simulink model "EvPowertrainController2EM"  (R2024a)
settings: configuration reference "VehicleFixed10ms" (kept outside this file)
model workspace (MAT data in the model file):
  CtrlVcuAccelPdlBpts = [0 0.8 1]
  CtrlVcuBattPnlty = 10000000
  CtrlVcuBattSOCBpts = [0 20 60 80 100]
  CtrlVcuCnstrntPnltyFctr = 10000000
  CtrlVcuEMPnlty = 100
  CtrlVcuEMTrqSplitGrid = 200
  CtrlVcuFallRate = -500
  CtrlVcuMaxAccelG = 1
  CtrlVcuMaxDecelG = -1.5
  CtrlVcuPwrDeltaPnlty = 50
  CtrlVcuPwrRatePnlty = [25 25 100]
  CtrlVcuRiseRate = 500
  CtrlVcuRoadMuEst = 0.8
  CtrlVcuSftyFctr = 0.9
  CtrlVcuTracPwrErrPnlty = 25
  CtrlVcuTrqVecBrkThresh = 0.01
  CtrlVcuTrqVecIGain = 0
  CtrlVcuTrqVecMinTrq = 25
  CtrlVcuTrqVecPGain = -2000
  CtrlVcuTrqVecSteerThresh = 0.349065850399
  CtrlVcuTrqVecVelThresh = 2.5
  N_P0 = 3
undefined symbols (not defined in the file): CtrlBcuTrlrBrkGain, CtrlVcuEvChrgLmtBpt, CtrlVcuEvRegenBrkCutOff, CtrlVcuEvRegenBrkSpdBpt, CtrlVcuEvSocBpt, eff, EnvGrvty, PlntBrkActrBoreFrnt, PlntBrkFrntBias, PlntBrkKinFricCffFrnt, PlntBrkNumPadsFrnt, PlntBrkPadMeanRadiusFrnt, PlntBrkPrsFctr, PlntBrkRearBias, PlntDiffrntl2Eff, PlntDiffrntl2Ratio, PlntDiffrntlEff, PlntDiffrntlRatio, PlntEM1EffTbl, PlntEM1Spd, PlntEM1SpdEff, PlntEM1Trq, PlntEM1TrqEff, PlntEM2EffTbl, PlntEM2Spd, PlntEM2SpdEff, PlntEM2Trq, PlntEM2TrqEff, PlntEM3EffTbl, PlntEM3Spd, PlntEM3SpdEff, PlntEM3Trq, PlntEM3TrqEff, PlntEMWhlGearEffFL, PlntEMWhlGearEffRL, PlntEMWhlGearRatioFL, PlntEMWhlGearRatioRL, PlntTransEffSpdBpt, PlntTransEffTbl, PlntTransEffTempBpt, PlntTransEffTrqBpt, PlntTransGearNumVect, PlntTransGearRatioVect, PlntVehCGHgtAxl, PlntVehDstCGFrntAxl, PlntVehDstCGRearAxl, PlntVehMass, PlntWhlLdRadius
libraries: simulink x16, autolibutils x2, slpidlib x2
(part 2 of 5)

== system EvPowertrainController2EM/Energy Management/Calculate Average EMSpd and Wheel Torque Curves for Front and Rear Axles/3EM Dual Front ==
  note: Calculate average speed
      | of EMs on axle
  note: Reflect EMTrq to WhlTrq
      | due to possible gearing
      | differences
  EMSpd : Inport
  Gear : Inport  Port=2
  EMTrq2WhlTrqFrnt : Subsystem  Variant=on  VariantControlMode=label  VariantControl=1  LabelModeActiveChoice=3
  EMTrq2WhlTrqRear : Subsystem  Variant=on  VariantControlMode=label  VariantControl=1  LabelModeActiveChoice=3
  Gain : Gain  Gain=1/2
  Maximum Torque Front Axle : Subsystem
  Maximum Torque Rear Axle : Subsystem
  Selector : Selector  InputPortWidth=3  IndexOptions=Index vector (dialog)  Indices=[1 2]  OutputSizes=1
  Selector1 : Selector  InputPortWidth=3  IndexOptions=Index vector (dialog)  Indices=[3]  OutputSizes=1
  Sum of Elements : Sum  Inputs=+
  Vector Concatenate : Concatenate
  Vector Concatenate1 : Concatenate
  EMAvgSpdVec : Outport
  WhlTrqMaxVec : Outport  Port=2
  wires:
  Selector/1 -> Sum of Elements/1
  EMSpd/1 -> Selector1/1, Selector/1
  Sum of Elements/1 -> Gain/1
  Maximum Torque Rear Axle/1(EMTrq) -> EMTrq2WhlTrqRear/2(EMTrqCmd)
  Maximum Torque Front Axle/1(EMTrq) -> EMTrq2WhlTrqFrnt/2(EMTrqCmd)
  Gain/1 -> Vector Concatenate1/1, EMTrq2WhlTrqFrnt/3(EMSpd), Maximum Torque Front Axle/1(EMSpd)
  Gear/1 -> EMTrq2WhlTrqRear/1(Gear), EMTrq2WhlTrqFrnt/1(Gear)
  Selector1/1 -> Maximum Torque Rear Axle/1(EMSpd), EMTrq2WhlTrqRear/3(EMSpd), Vector Concatenate1/2
  EMTrq2WhlTrqRear/1(WhlMotTrq) -> Vector Concatenate/2
  EMTrq2WhlTrqFrnt/1(WhlMotTrq) -> Vector Concatenate/1
  Vector Concatenate/1 -> WhlTrqMaxVec/1
  Vector Concatenate1/1 -> EMAvgSpdVec/1

== system EvPowertrainController2EM/Energy Management/Calculate Average EMSpd and Wheel Torque Curves for Front and Rear Axles/3EM Dual Rear ==
  note: Calculate average speed
      | of EMs on axle
  note: Reflect EMTrq to WhlTrq
      | due to possible gearing
      | differences
  EMSpd : Inport
  Gear : Inport  Port=2
  EMTrq2WhlTrqFrnt : Subsystem  Variant=on  VariantControlMode=label  VariantControl=1  LabelModeActiveChoice=3
  EMTrq2WhlTrqRear : Subsystem  Variant=on  VariantControlMode=label  VariantControl=1  LabelModeActiveChoice=3
  Gain : Gain  Gain=1/2
  Maximum Torque Front Axle : Subsystem
  Maximum Torque Rear Axle : Subsystem
  Selector : Selector  InputPortWidth=3  IndexOptions=Index vector (dialog)  Indices=[2 3]  OutputSizes=1
  Selector1 : Selector  InputPortWidth=3  IndexOptions=Index vector (dialog)  Indices=[1]  OutputSizes=1
  Sum of Elements : Sum  Inputs=+
  Vector Concatenate : Concatenate
  Vector Concatenate1 : Concatenate
  EMAvgSpdVec : Outport
  WhlTrqMaxVec : Outport  Port=2
  wires:
  Sum of Elements/1 -> Gain/1
  EMSpd/1 -> Selector1/1, Selector/1
  Selector/1 -> Sum of Elements/1
  EMTrq2WhlTrqRear/1(WhlMotTrq) -> Vector Concatenate/2
  Gain/1 -> Vector Concatenate1/2, EMTrq2WhlTrqRear/3(EMSpd), Maximum Torque Rear Axle/1(EMSpd)
  Maximum Torque Rear Axle/1(EMTrq) -> EMTrq2WhlTrqRear/2(EMTrqCmd)
  Maximum Torque Front Axle/1(EMTrq) -> EMTrq2WhlTrqFrnt/2(EMTrqCmd)
  Selector1/1 -> Vector Concatenate1/1, EMTrq2WhlTrqFrnt/3(EMSpd), Maximum Torque Front Axle/1(EMSpd)
  Gear/1 -> EMTrq2WhlTrqFrnt/1(Gear), EMTrq2WhlTrqRear/1(Gear)
  EMTrq2WhlTrqFrnt/1(WhlMotTrq) -> Vector Concatenate/1
  Vector Concatenate/1 -> WhlTrqMaxVec/1
  Vector Concatenate1/1 -> EMAvgSpdVec/1

== system EvPowertrainController2EM/Energy Management/Calculate Average EMSpd and Wheel Torque Curves for Front and Rear Axles/4EM ==
  note: Calculate average speed
      | of EMs on axle
  note: Reflect EMTrq to WhlTrq
      | due to possible gearing
      | differences
  EMSpd : Inport
  Gear : Inport  Port=2
  EMTrq2WhlTrqFrnt : Subsystem  Variant=on  VariantControlMode=label  VariantControl=1  LabelModeActiveChoice=3
  EMTrq2WhlTrqRear : Subsystem  Variant=on  VariantControlMode=label  VariantControl=1  LabelModeActiveChoice=3
  Gain : Gain  Gain=1/2
  Gain1 : Gain  Gain=1/2
  Maximum Torque Front Axle : Subsystem
  Maximum Torque Rear Axle : Subsystem
  Selector : Selector  InputPortWidth=4  IndexOptions=Index vector (dialog)  Indices=[3 4]  OutputSizes=1
  Selector1 : Selector  InputPortWidth=4  IndexOptions=Index vector (dialog)  Indices=[1 2]  OutputSizes=1
  Sum of Elements : Sum  Inputs=+
  Sum of Elements1 : Sum  Inputs=+
  Vector Concatenate : Concatenate
  Vector Concatenate1 : Concatenate
  EMAvgSpdVec : Outport
  WhlTrqMaxVec : Outport  Port=2
  wires:
  Selector/1 -> Sum of Elements/1
  Selector1/1 -> Sum of Elements1/1
  EMSpd/1 -> Selector/1, Selector1/1
  Sum of Elements/1 -> Gain/1
  Sum of Elements1/1 -> Gain1/1
  EMTrq2WhlTrqRear/1(WhlMotTrq) -> Vector Concatenate/2
  Maximum Torque Front Axle/1(EMTrq) -> EMTrq2WhlTrqFrnt/2(EMTrqCmd)
  Maximum Torque Rear Axle/1(EMTrq) -> EMTrq2WhlTrqRear/2(EMTrqCmd)
  Gain1/1 -> Vector Concatenate1/1, EMTrq2WhlTrqFrnt/3(EMSpd), Maximum Torque Front Axle/1(EMSpd)
  EMTrq2WhlTrqFrnt/1(WhlMotTrq) -> Vector Concatenate/1
  Gear/1 -> EMTrq2WhlTrqRear/1(Gear), EMTrq2WhlTrqFrnt/1(Gear)
  Gain/1 -> Vector Concatenate1/2, Maximum Torque Rear Axle/1(EMSpd), EMTrq2WhlTrqRear/3(EMSpd)
  Vector Concatenate/1 -> WhlTrqMaxVec/1
  Vector Concatenate1/1 -> EMAvgSpdVec/1

== system EvPowertrainController2EM/Energy Management/Control Domain /Front Axle EM Torque Vector ==
  EMAvgSpdVec : Inport
  2EM or 3EM Dual Rear : Subsystem  VariantControl=2EM or 3EM Dual Rear
  3EM Dual Front or 4EM : Subsystem  VariantControl=3EM Dual Front or 4EM
  WhlEMFrntVecPos : Outport
  WhlEMFrntVecNeg : Outport  Port=2

== system EvPowertrainController2EM/Energy Management/Control Domain /Rear Axle EM Torque Vector ==
  EMAvgSpdVec : Inport
  2EM or 3EM Dual Front : Subsystem  VariantControl=2EM or 3EM Dual Front
  3EM Dual Rear or 4EM : Subsystem  VariantControl=3EM Dual Rear or 4EM
  WhlEMRearVecPos : Outport
  WhlEMRearVecNeg : Outport  Port=2

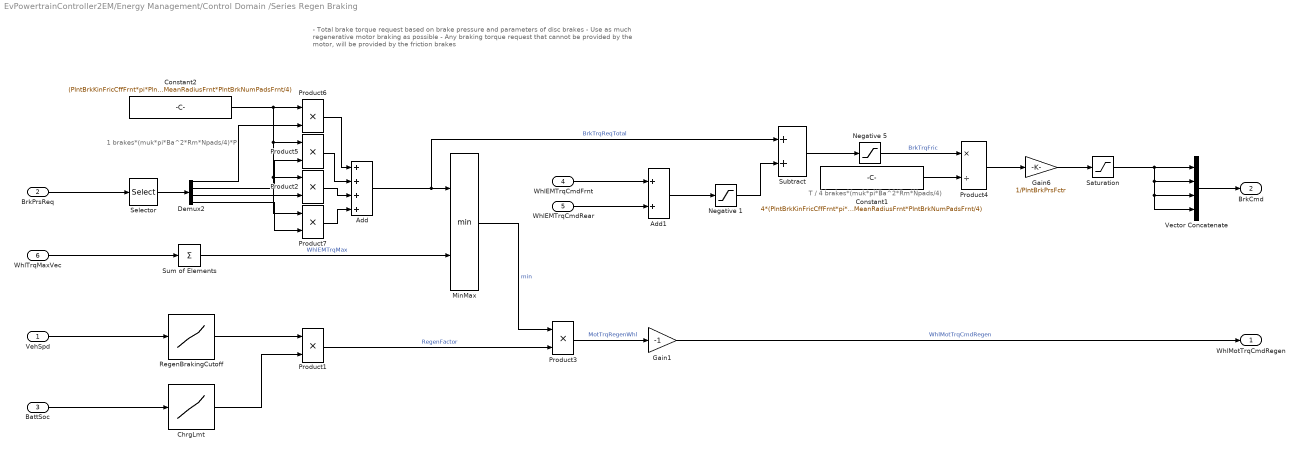
== system EvPowertrainController2EM/Energy Management/Control Domain /Series Regen Braking ==
  note: - Total brake torque request based on brake pressure and parameters of disc brakes
      | - Use as much regenerative motor braking as possible
      | - Any braking torque request that cannot be provided by the motor, will be provided by the friction brakes
  note: T / 4 brakes*(muk*pi*Ba^2*Rm*Npads/4)
  note: 1 brakes*(muk*pi*Ba^2*Rm*Npads/4)*P
  VehSpd : Inport
  "BrkPrsReq " : Inport  Port=2
  BattSoc : Inport  Port=3
  WhlEMTrqCmdFrnt : Inport  Port=4
  WhlEMTrqCmdRear : Inport  Port=5
  WhlTrqMaxVec : Inport  Port=6
  Add : Sum  Inputs=++++
  Add1 : Sum
  ChrgLmt : Lookup_n-D  NumberOfTableDimensions=1  BreakpointsForDimension1=CtrlVcuEvSocBpt  Table=CtrlVcuEvChrgLmtBpt  ExtrapMethod=Clip  UseLastTableValue=on  InternalRulePriority=Speed  RndMeth=Simplest
  Constant1 : Constant  Value=4*(PlntBrkKinFricCffFrnt*pi*PlntBrkActrBoreFrnt^2*PlntBrkPadMeanRadiusFrnt*PlntBrkNumPadsFrnt/4)
  Constant2 : Constant  Value=(PlntBrkKinFricCffFrnt*pi*PlntBrkActrBoreFrnt^2*PlntBrkPadMeanRadiusFrnt*PlntBrkNumPadsFrnt/4)
  Demux2 : Demux
  Gain1 : Gain  Gain=-1
  Gain6 : Gain  Gain=1/PlntBrkPrsFctr
  MinMax : MinMax  Inputs=2
  Negative 1 : Saturate  UpperLimit=0  LowerLimit=-inf
  Negative 5 : Saturate  UpperLimit=inf  LowerLimit=0
  Product{1..3,5..7} (6 alike) : Product
  Product4 : Product  Inputs=*/
  RegenBrakingCutoff : Lookup_n-D  NumberOfTableDimensions=1  BreakpointsForDimension1=CtrlVcuEvRegenBrkSpdBpt  Table=CtrlVcuEvRegenBrkCutOff  ExtrapMethod=Clip  UseLastTableValue=on  InternalRulePriority=Speed  RndMeth=Simplest
  Saturation : Saturate  UpperLimit=1  LowerLimit=0
  Selector : Selector  InputPortWidth=4  IndexOptions=Index vector (dialog)  Indices=[1 2 3 4]  OutputSizes=1
  Subtract : Sum
  Sum of Elements : Sum  Inputs=+
  Vector Concatenate : Concatenate  NumInputs=4
  " WhlMotTrqCmdRegen" : Outport  VectorParamsAs1DForOutWhenUnconnected=off
  " BrkCmd" : Outport  Port=2  VectorParamsAs1DForOutWhenUnconnected=off
  wires:
  Constant1/1 -> Product4/2
  MinMax/1 -> Product3/1  "min"
  ChrgLmt/1 -> Product1/2
  VehSpd/1 -> RegenBrakingCutoff/1
  RegenBrakingCutoff/1 -> Product1/1
  Product1/1 -> Product3/2  "RegenFactor"
  Subtract/1 -> Negative 5/1
  BattSoc/1 -> ChrgLmt/1
  Negative 5/1 -> Product4/1  "BrkTrqFric"
  Sum of Elements/1 -> MinMax/2  "WhlEMTrqMax"
  Demux2/2 -> Product5/2
  Demux2/1 -> Product6/2
  Selector/1 -> Demux2/1
  Product6/1 -> Add/1
  Product5/1 -> Add/2
  Add/1 -> Subtract/1, MinMax/1  "BrkTrqReqTotal"
  "BrkPrsReq "/1 -> Selector/1
  Vector Concatenate/1 -> " BrkCmd"/1
  Gain6/1 -> Saturation/1
  Product4/1 -> Gain6/1
  Saturation/1 -> Vector Concatenate/3, Vector Concatenate/4, Vector Concatenate/2, Vector Concatenate/1
  WhlTrqMaxVec/1 -> Sum of Elements/1
  Gain1/1 -> " WhlMotTrqCmdRegen"/1  "WhlMotTrqCmdRegen"
  Product3/1 -> Gain1/1  "MotTrqRegenWhl"
  Add1/1 -> Negative 1/1
  Negative 1/1 -> Subtract/2
  Product2/1 -> Add/3
  Product7/1 -> Add/4
  Demux2/3 -> Product2/2
  Demux2/4 -> Product7/2
  Constant2/1 -> Product7/1, Product2/1, Product5/1, Product6/1
  WhlEMTrqCmdFrnt/1 -> Add1/1
  WhlEMTrqCmdRear/1 -> Add1/2

== system EvPowertrainController2EM/Energy Management/Convert Whl to EMTrq Vector/2EM ==
  WhlEMTrqCmdFrnt : Inport
  WhlEMTrqCmdRear : Inport  Port=2
  EMAvgSpdVec : Inport  Port=3
  Diff Eta : Subsystem
  Diff Eta1 : Subsystem
  Divide1 : Product  Inputs=/*
  Divide2 : Product  Inputs=/*
  Gain1 : Gain  Gain=1/PlntDiffrntl2Ratio
  Gain3 : Gain  Gain=1/PlntDiffrntlRatio
  Selector : Selector  InputPortWidth=2  IndexOptions=Index vector (dialog)  Indices=[1]  OutputSizes=1
  Selector1 : Selector  InputPortWidth=2  IndexOptions=Index vector (dialog)  Indices=[2]  OutputSizes=1
  Unit Delay : UnitDelay  SampleTime=-1  HasFrameUpgradeWarning=on
  Unit Delay1 : UnitDelay  SampleTime=-1  HasFrameUpgradeWarning=on
  Vector Concatenate1 : Concatenate
  EMTrqCmd : Outport
  wires:
  WhlEMTrqCmdRear/1 -> Gain1/1
  Gain3/1 -> Divide2/2
  Divide2/1 -> Vector Concatenate1/1, Unit Delay/1
  WhlEMTrqCmdFrnt/1 -> Gain3/1
  Selector/1 -> Diff Eta/1(SpdIn)
  Unit Delay/1 -> Diff Eta/2(TrqIn)
  Diff Eta/1(eta) -> Divide2/1
  Diff Eta1/1(eta) -> Divide1/1
  Unit Delay1/1 -> Diff Eta1/2(TrqIn)
  Divide1/1 -> Unit Delay1/1, Vector Concatenate1/2
  Gain1/1 -> Divide1/2
  EMAvgSpdVec/1 -> Selector1/1, Selector/1
  Selector1/1 -> Diff Eta1/1(SpdIn)
  Vector Concatenate1/1 -> EMTrqCmd/1

== system EvPowertrainController2EM/Energy Management/Convert Whl to EMTrq Vector/3EM Dual Front ==
  WhlEMTrqCmdFrnt : Inport
  WhlEMTrqCmdRear : Inport  Port=2
  EMAvgSpdVec : Inport  Port=3
  Diff Eta : Subsystem
  Divide1 : Product  Inputs=/*
  Divide2 : Product  Inputs=/*
  Dual EMs : Gain  Gain=1/2
  Gain1 : Gain  Gain=1/PlntDiffrntl2Ratio
  Gain3 : Gain  Gain=1/PlntEMWhlGearRatioFL
  Gear Eta : Subsystem
  Selector : Selector  InputPortWidth=2  IndexOptions=Index vector (dialog)  Indices=[1]  OutputSizes=1
  Selector1 : Selector  InputPortWidth=2  IndexOptions=Index vector (dialog)  Indices=[2]  OutputSizes=1
  Unit Delay : UnitDelay  SampleTime=-1  HasFrameUpgradeWarning=on
  Unit Delay1 : UnitDelay  SampleTime=-1  HasFrameUpgradeWarning=on
  Vector Concatenate : Concatenate  NumInputs=3
  EMTrqCmd : Outport
  wires:
  Selector1/1 -> Diff Eta/1(SpdIn)
  EMAvgSpdVec/1 -> Selector/1, Selector1/1
  Gain1/1 -> Divide1/2
  Unit Delay1/1 -> Diff Eta/2(TrqIn)
  Diff Eta/1(eta) -> Divide1/1
  Gear Eta/1(eta) -> Divide2/1
  Unit Delay/1 -> Gear Eta/2(TrqIn)
  Selector/1 -> Gear Eta/1(SpdIn)
  WhlEMTrqCmdFrnt/1 -> Dual EMs/1
  Gain3/1 -> Divide2/2
  WhlEMTrqCmdRear/1 -> Gain1/1
  Divide1/1 -> Vector Concatenate/3, Unit Delay1/1
  Vector Concatenate/1 -> EMTrqCmd/1
  Divide2/1 -> Vector Concatenate/1, Vector Concatenate/2, Unit Delay/1
  Dual EMs/1 -> Gain3/1

== system EvPowertrainController2EM/Energy Management/Convert Whl to EMTrq Vector/3EM Dual Rear ==
  WhlEMTrqCmdFrnt : Inport
  WhlEMTrqCmdRear : Inport  Port=2
  EMAvgSpdVec : Inport  Port=3
  Diff Eta : Subsystem
  Divide1 : Product  Inputs=/*
  Divide2 : Product  Inputs=/*
  Dual EMs : Gain  Gain=1/2
  Gain1 : Gain  Gain=1/PlntEMWhlGearRatioRL
  Gain3 : Gain  Gain=1/PlntDiffrntlRatio
  Gear Eta : Subsystem
  Selector : Selector  InputPortWidth=2  IndexOptions=Index vector (dialog)  Indices=[1]  OutputSizes=1
  Selector1 : Selector  InputPortWidth=2  IndexOptions=Index vector (dialog)  Indices=[2]  OutputSizes=1
  Unit Delay : UnitDelay  SampleTime=-1  HasFrameUpgradeWarning=on
  Unit Delay1 : UnitDelay  SampleTime=-1  HasFrameUpgradeWarning=on
  Vector Concatenate : Concatenate  NumInputs=3
  EMTrqCmd : Outport
  wires:
  WhlEMTrqCmdFrnt/1 -> Gain3/1
  Divide2/1 -> Unit Delay/1, Vector Concatenate/1
  Vector Concatenate/1 -> EMTrqCmd/1
  Divide1/1 -> Unit Delay1/1, Vector Concatenate/2, Vector Concatenate/3
  WhlEMTrqCmdRear/1 -> Dual EMs/1
  Gain3/1 -> Divide2/2
  Selector/1 -> Diff Eta/1(SpdIn)
  Unit Delay/1 -> Diff Eta/2(TrqIn)
  Diff Eta/1(eta) -> Divide2/1
  Gear Eta/1(eta) -> Divide1/1
  Unit Delay1/1 -> Gear Eta/2(TrqIn)
  Gain1/1 -> Divide1/2
  EMAvgSpdVec/1 -> Selector1/1, Selector/1
  Selector1/1 -> Gear Eta/1(SpdIn)
  Dual EMs/1 -> Gain1/1

== system EvPowertrainController2EM/Energy Management/Convert Whl to EMTrq Vector/4EM ==
  WhlEMTrqCmdFrnt : Inport
  WhlEMTrqCmdRear : Inport  Port=2
  EMAvgSpdVec : Inport  Port=3
  Divide1 : Product  Inputs=/*
  Divide2 : Product  Inputs=/*
  Dual EMs : Gain  Gain=1/2
  Dual EMs1 : Gain  Gain=1/2
  Gain1 : Gain  Gain=1/PlntEMWhlGearRatioRL
  Gain3 : Gain  Gain=1/PlntEMWhlGearRatioFL
  Gear Eta : Subsystem
  Gear Eta1 : Subsystem
  Selector : Selector  InputPortWidth=2  IndexOptions=Index vector (dialog)  Indices=[1]  OutputSizes=1
  Selector1 : Selector  InputPortWidth=2  IndexOptions=Index vector (dialog)  Indices=[2]  OutputSizes=1
  Unit Delay : UnitDelay  SampleTime=-1  HasFrameUpgradeWarning=on
  Unit Delay1 : UnitDelay  SampleTime=-1  HasFrameUpgradeWarning=on
  Vector Concatenate : Concatenate  NumInputs=4
  EMTrqCmd : Outport
  wires:
  Dual EMs1/1 -> Gain1/1
  Selector1/1 -> Gear Eta1/1(SpdIn)
  EMAvgSpdVec/1 -> Selector/1, Selector1/1
  Gain1/1 -> Divide1/2
  Unit Delay1/1 -> Gear Eta1/2(TrqIn)
  Gear Eta1/1(eta) -> Divide1/1
  Gear Eta/1(eta) -> Divide2/1
  Unit Delay/1 -> Gear Eta/2(TrqIn)
  Selector/1 -> Gear Eta/1(SpdIn)
  Gain3/1 -> Divide2/2
  WhlEMTrqCmdRear/1 -> Dual EMs1/1
  Divide1/1 -> Vector Concatenate/4, Vector Concatenate/3, Unit Delay1/1
  Vector Concatenate/1 -> EMTrqCmd/1
  Divide2/1 -> Vector Concatenate/2, Unit Delay/1, Vector Concatenate/1
  WhlEMTrqCmdFrnt/1 -> Dual EMs/1
  Dual EMs/1 -> Gain3/1

== system EvPowertrainController2EM/Energy Management/Hamiltonian computation and minimization/Pwr Rate Limit ==
  note: This table helps reduce rapid oscillations in torque
      | that can occur when operating at WOT conditions which
      | can result in the torque being limited by the BMS.
  note: There could be instances where an mot trq command produces the minimum cost, but differs greatly from the previously selected mot trq.
      |
      | This function will calculate the difference in power between the current mot power vector and the previously selected mot pwr.  This term is added to the total cost function, and will help limit the rate at which the mot power (and torque) can change from time step to time step.
  note: Alternative to using
      | abs funciton
  WhlEMTrqVec : Inport
  WhlSpd : Inport  Port=2
  PrevWhlEMTrqCmd : Inport  Port=3
  AccelPdl : Inport  Port=4
  1-D Lookup Table : Lookup_n-D  NumberOfTableDimensions=1  BreakpointsForDimension1=CtrlVcuAccelPdlBpts  BeginIndexSearchUsingPreviousIndexResult=on  Table=CtrlVcuPwrRatePnlty  ExtrapMethod=Clip  UseLastTableValue=on  InternalRulePriority=Speed  RndMeth=Simplest
  Product{,1,6..7} (4 alike) : Product
  Sqrt1 : Sqrt
  Subtract : Sum  Inputs=+-
  W2kW : Gain  Gain=1/1000
  EMPwrDelta : Outport  VectorParamsAs1DForOutWhenUnconnected=off
  wires:
  Product7/1 -> Sqrt1/1
  Product6/1 -> Subtract/1  "PwrVec"
  Product1/1 -> Subtract/2  "PrevPwr"
  WhlSpd/1 -> Product6/2, Product1/1
  PrevWhlEMTrqCmd/1 -> Product1/2
  Subtract/1 -> Product7/1, Product7/2
  Sqrt1/1 -> W2kW/1
  WhlEMTrqVec/1 -> Product6/1
  W2kW/1 -> Product/1
  Product/1 -> EMPwrDelta/1
  AccelPdl/1 -> 1-D Lookup Table/1
  1-D Lookup Table/1 -> Product/2

== system EvPowertrainController2EM/Energy Management/Powertrain Constraints /Battery Constraint ==
  EMPwrElecVec : Inport
  BattVin : Inport  Port=2
  BattPwrDisChrgLmt : Inport  Port=3
  "BattPwrChrgLmt " : Inport  Port=4
  Electrical Current : Subsystem
  Logical Operator : Logic  Operator=OR  Inputs=4  AllPortsSameDT=off  OutDataTypeStr=boolean
  Power Limit Calculations : Subsystem
  Relational Operator : RelationalOperator  Operator=>  OutDataTypeStr=boolean  InputSameDT=off
  Relational Operator1 : RelationalOperator  Operator=>  OutDataTypeStr=boolean  InputSameDT=off
  Relational Operator2 : RelationalOperator  Operator=<  OutDataTypeStr=boolean  InputSameDT=off
  Relational Operator3 : RelationalOperator  Operator=<  OutDataTypeStr=boolean  InputSameDT=off
  Saturation Dynamic : simulink/Discontinuities/Saturation Dynamic  OutMin=[]  OutMax=[]  OutDataTypeStr=Inherit: Same as second input  OutDataType=fixdt(1, 16)  OutScaling=2^-10  DoSatur=off
  InfeasibleBatt : Outport  VectorParamsAs1DForOutWhenUnconnected=off
  BattCurr : Outport  Port=2  VectorParamsAs1DForOutWhenUnconnected=off
  BattV : Outport  Port=3  VectorParamsAs1DForOutWhenUnconnected=off
  wires:
  Saturation Dynamic/1 -> BattCurr/1
  Logical Operator/1 -> InfeasibleBatt/1
  Relational Operator1/1 -> Logical Operator/3
  EMPwrElecVec/1 -> Relational Operator1/1, Relational Operator2/1, Electrical Current/2(EMPwrElecVec)
  Relational Operator2/1 -> Logical Operator/4
  Power Limit Calculations/3(BattPwrDischrgLmt) -> Relational Operator1/2
  Power Limit Calculations/4(BattPwrChrgLmt) -> Relational Operator2/2
  BattVin/1 -> Electrical Current/1(BattV), Power Limit Calculations/3(BattV_in), BattV/1
  [DischrgLmt] -> Saturation Dynamic/1
  [ChrgLmt] -> Saturation Dynamic/3
  Relational Operator/1 -> Logical Operator/1
  Electrical Current/1(BatteryAmp) -> Relational Operator3/1, Relational Operator/1, Saturation Dynamic/2
  "BattPwrChrgLmt "/1 -> Power Limit Calculations/2("BattPwrChrgLmt ")
  BattPwrDisChrgLmt/1 -> Power Limit Calculations/1(BattPwrDisChrgLmt)
  Power Limit Calculations/1(BattCurrDischrgLmt) -> [DischrgLmt]
  Power Limit Calculations/2(BattCurrChrgLmt) -> [ChrgLmt]
  [DischrgLmt] -> Relational Operator/2
  [ChrgLmt] -> Relational Operator3/2
  Relational Operator3/1 -> Logical Operator/2

== system EvPowertrainController2EM/Energy Management/Powertrain Constraints /EM Constraint Front ==
  WhlTrqCmd : Inport
  EMAvgSpdVec : Inport  Port=2
  WhlEMTrqSplitVecFrnt : Inport  Port=3
  WhlTrqMaxVec : Inport  Port=4
  Maximum Torque : Subsystem  VariantControl=2EM
  Tabular Power Loss Data : Subsystem  Variant=on  VariantControlMode=label  VariantControl=Choice  LabelModeActiveChoice=2EM or 3EM Dual Rear
  Wheel Torque Saturation for Max g Rates : Subsystem
  WhlEMTrqSatVec : Outport  VectorParamsAs1DForOutWhenUnconnected=off
  InfeasibleEMVec : Outport  Port=2  VectorParamsAs1DForOutWhenUnconnected=off
  EMPwrElecVec : Outport  Port=3  VectorParamsAs1DForOutWhenUnconnected=off
  wires:
  WhlTrqMaxVec/1 -> Maximum Torque/3(WhlTrqMaxVec)
  Tabular Power Loss Data/1(EMPwrElecVec) -> EMPwrElecVec/1
  Maximum Torque/2(InfeasibleEMVec) -> InfeasibleEMVec/1
  Wheel Torque Saturation for Max g Rates/1(tqOut) -> Maximum Torque/2(WhlEMTrqSplitVecFrnt)
  WhlTrqCmd/1 -> Wheel Torque Saturation for Max g Rates/1(WhlTrqCmd), Maximum Torque/1(WhlTrqCmd)
  EMAvgSpdVec/1 -> Tabular Power Loss Data/1(EMAvgSpdVec)
  Maximum Torque/1(WhlEMTrqSatVec) -> Tabular Power Loss Data/2(WhlEMTrqSatVec), WhlEMTrqSatVec/1
  WhlEMTrqSplitVecFrnt/1 -> Wheel Torque Saturation for Max g Rates/2(Tqin)

== system EvPowertrainController2EM/Energy Management/Powertrain Constraints /EM Constraint Rear ==
  WhlTrqCmd : Inport
  EMAvgSpdVec : Inport  Port=2
  WhlEMTrqSplitVecRear : Inport  Port=3
  WhlTrqMaxVec : Inport  Port=4
  Maximum Torque : Subsystem  VariantControl=2EM
  Tabular Power Loss Data : Subsystem  Variant=on  VariantControlMode=label  VariantControl=Choice  LabelModeActiveChoice=2EM
  Wheel Torque Saturation for Max g Rates : Subsystem
  WhlEMTrqSatVec : Outport  VectorParamsAs1DForOutWhenUnconnected=off
  InfeasibleEMVec : Outport  Port=2  VectorParamsAs1DForOutWhenUnconnected=off
  EMPwrElecVec : Outport  Port=3  VectorParamsAs1DForOutWhenUnconnected=off
  wires:
  Maximum Torque/1(WhlEMTrqSatVec) -> WhlEMTrqSatVec/1, Tabular Power Loss Data/2(WhlEMTrqSatVec)
  EMAvgSpdVec/1 -> Tabular Power Loss Data/1(EMAvgSpdVec)
  WhlTrqCmd/1 -> Wheel Torque Saturation for Max g Rates/1(WhlTrqCmd), Maximum Torque/1(WhlTrqCmd)
  Wheel Torque Saturation for Max g Rates/1(tqOut) -> Maximum Torque/2(WhlEMTrqSplitVecRear)
  Maximum Torque/2(InfeasibleEMVec) -> InfeasibleEMVec/1
  Tabular Power Loss Data/1(EMPwrElecVec) -> EMPwrElecVec/1
  WhlTrqMaxVec/1 -> Maximum Torque/3(WhlTrqMaxVec)
  WhlEMTrqSplitVecRear/1 -> Wheel Torque Saturation for Max g Rates/2(Tqin)

== system EvPowertrainController2EM/Energy Management/Powertrain Constraints /Wheel Torque Vector Logic ==
  note: Traction will start with Rear EM Torque Split Vector than calculate Front EM Torque Split
      |
      | Regen will start with Front EM Torque Split Vector than calculate Rear EM Torque Split
  WhlTrqCmd : Inport
  WhlEMTrqSplitVecFrnt : Inport  Port=2
  WhlEMTrqSplitVecRear : Inport  Port=3
  WhlEMTrqSatVecRear : Inport  Port=4
  WhlEMTrqSatVecFrnt : Inport  Port=5
  If : If  IfExpression=u1 >= 0
  Merge : Merge
  Merge1 : Merge
  Regen : Subsystem
  Traction : Subsystem
  WhlEMTrqSplitVecFrnt1 : Outport
  WhlEMTrqSplitVecRear1 : Outport  Port=2
  wires:
  WhlTrqCmd/1 -> If/1, Regen/1(WhlTrqCmd), Traction/1(WhlTrqCmd)
  WhlEMTrqSatVecRear/1 -> Traction/2(WhlEMTrqSatVecRear)
  WhlEMTrqSplitVecFrnt/1 -> Traction/3(WhlEMTrqSplitVecFrnt), Regen/3(WhlEMTrqSplitVecFrnt)
  WhlEMTrqSplitVecRear/1 -> Traction/4(WhlEMTrqSplitVecRear), Regen/4(WhlEMTrqSplitVecRear)
  Traction/1(WhlEMTrqSplitVecFrnt1) -> Merge/1
  Traction/2(WhlEMTrqSplitVecRear1) -> Merge1/1
  If/1 -> Traction/Action
  If/2 -> Regen/Action
  Merge/1 -> WhlEMTrqSplitVecFrnt1/1
  Merge1/1 -> WhlEMTrqSplitVecRear1/1
  Regen/1(WhlEMTrqSplitVecFrnt1) -> Merge/2
  Regen/2(WhlEMTrqSplitVecRear1) -> Merge1/2
  WhlEMTrqSatVecFrnt/1 -> Regen/2(WhlEMTrqSatVecFrnt)

== system EvPowertrainController2EM/Torque Vectoring/3EM/Create EMTrq Vector ==
  EMTrqSplit : Inport
  EMTrqCmd : Inport  Port=2
  3EMDualFront : Subsystem  VariantControl=3EMDualFront
  3EMDualRear : Subsystem  VariantControl=3EMDualRear
  EMTrqCmdFinal : Outport

== system EvPowertrainController2EM/Torque Vectoring/3EM/EMTrq ==
  EMSpd : Inport
  EMTrqCmd : Inport  Port=2
  3EMDualFront : Subsystem  VariantControl=3EMDualFront
  3EMDualRear : Subsystem  VariantControl=3EMDualRear
  EMTrqMax : Outport
  EMTrqL : Outport  Port=2
  EMTrqR : Outport  Port=3

== system EvPowertrainController2EM/Torque Vectoring/4EM/EMTrq ==
  EMSpd : Inport
  EMTrqCmd : Inport  Port=2
  Dual Front : Subsystem  VariantControl=3EMDualFront
  Dual Rear : Subsystem  VariantControl=3EMDualRear
  EMTrqMaxFrnt : Outport
  EMTrqFL : Outport  Port=2
  EMTrqFR : Outport  Port=3
  EMTrqMaxRear : Outport  Port=4
  EMTrqRL : Outport  Port=5
  EMTrqRR : Outport  Port=6
  wires:
  EMTrqCmd/1 -> Dual Rear/2(EMTrqCmd), Dual Front/2(EMTrqCmd)
  Dual Front/1(EMTrqMaxFrnt) -> EMTrqMaxFrnt/1
  EMSpd/1 -> Dual Rear/1(EMSpd), Dual Front/1(EMSpd)
  Dual Rear/1(EMTrqMaxRear) -> EMTrqMaxRear/1
  Dual Front/3(EMTrqFR) -> EMTrqFR/1
  Dual Front/2(EMTrqFL) -> EMTrqFL/1
  Dual Rear/3(EMTrqRR) -> EMTrqRR/1
  Dual Rear/2(EMTrqRL) -> EMTrqRL/1

== system EvPowertrainController2EM/Accel Pedal to Traction Wheel Torque Request/EM2WhlTrq/2EM/EMTrq2WhlTrqFrnt ==
  Gear : Inport
  EMTrqCmd : Inport  Port=2
  EMSpd : Inport  Port=3
  No Transmission : Subsystem  VariantControl=3
  Transmission : Subsystem  VariantControl=1
  WhlMotTrq : Outport

== system EvPowertrainController2EM/Accel Pedal to Traction Wheel Torque Request/EM2WhlTrq/2EM/EMTrq2WhlTrqRear ==
  Gear : Inport
  EMTrqCmd : Inport  Port=2
  EMSpd : Inport  Port=3
  No Transmission : Subsystem  VariantControl=3
  Transmission : Subsystem  VariantControl=1
  WhlMotTrq : Outport

== system EvPowertrainController2EM/Accel Pedal to Traction Wheel Torque Request/EM2WhlTrq/2EM/Maximum Torque Front Axle ==
  EMSpd : Inport
  MaxEMTrqVsSpd : Lookup_n-D  NumberOfTableDimensions=1  BreakpointsForDimension1=PlntEM1Spd  Table=PlntEM1Trq  ExtrapMethod=Clip  UseLastTableValue=on  InternalRulePriority=Speed  OutDataTypeStr=Inherit: Inherit from 'Table data'  RndMeth=Simplest
  EMTrq : Outport  VectorParamsAs1DForOutWhenUnconnected=off
  wires:
  MaxEMTrqVsSpd/1 -> EMTrq/1
  EMSpd/1 -> MaxEMTrqVsSpd/1

== system EvPowertrainController2EM/Accel Pedal to Traction Wheel Torque Request/EM2WhlTrq/2EM/Maximum Torque Rear Axle ==
  EMSpd : Inport
  MaxEMTrqVsSpd : Lookup_n-D  NumberOfTableDimensions=1  BreakpointsForDimension1=PlntEM2Spd  Table=PlntEM2Trq  ExtrapMethod=Clip  UseLastTableValue=on  InternalRulePriority=Speed  OutDataTypeStr=Inherit: Inherit from 'Table data'  RndMeth=Simplest
  EMTrq : Outport  VectorParamsAs1DForOutWhenUnconnected=off
  wires:
  MaxEMTrqVsSpd/1 -> EMTrq/1
  EMSpd/1 -> MaxEMTrqVsSpd/1

== system EvPowertrainController2EM/Accel Pedal to Traction Wheel Torque Request/EM2WhlTrq/2EM/VehSpd2EMSpd ==
  Gear : Inport
  VehSpd : Inport  Port=2
  No Transmission : Subsystem  VariantControl=3
  Transmission : Subsystem  VariantControl=1
  EMSpdFrntAxl : Outport
  EMSpdRearAxl : Outport  Port=2

== system EvPowertrainController2EM/Accel Pedal to Traction Wheel Torque Request/EM2WhlTrq/3EM Dual Front/EMTrq2WhlTrqFrnt ==
  Gear : Inport
  EMTrqCmd : Inport  Port=2
  EMSpd : Inport  Port=3
  No Transmission : Subsystem  VariantControl=3
  Transmission : Subsystem  VariantControl=1
  WhlMotTrq : Outport

== system EvPowertrainController2EM/Accel Pedal to Traction Wheel Torque Request/EM2WhlTrq/3EM Dual Front/EMTrq2WhlTrqRear ==
  Gear : Inport
  EMTrqCmd : Inport  Port=2
  EMSpd : Inport  Port=3
  No Transmission : Subsystem  VariantControl=3
  Transmission : Subsystem  VariantControl=1
  WhlMotTrq : Outport

== system EvPowertrainController2EM/Accel Pedal to Traction Wheel Torque Request/EM2WhlTrq/3EM Dual Front/Maximum Torque Front Axle ==
  EMSpd : Inport
  MaxEMTrqVsSpd : Lookup_n-D  NumberOfTableDimensions=1  BreakpointsForDimension1=PlntEM1Spd  Table=PlntEM1Trq  ExtrapMethod=Clip  UseLastTableValue=on  InternalRulePriority=Speed  OutDataTypeStr=Inherit: Inherit from 'Table data'  RndMeth=Simplest
  EMTrq : Outport  VectorParamsAs1DForOutWhenUnconnected=off
  wires:
  EMSpd/1 -> MaxEMTrqVsSpd/1
  MaxEMTrqVsSpd/1 -> EMTrq/1

== system EvPowertrainController2EM/Accel Pedal to Traction Wheel Torque Request/EM2WhlTrq/3EM Dual Front/Maximum Torque Rear Axle ==
  EMSpd : Inport
  MaxEMTrqVsSpd : Lookup_n-D  NumberOfTableDimensions=1  BreakpointsForDimension1=PlntEM3Spd  Table=PlntEM3Trq  ExtrapMethod=Clip  UseLastTableValue=on  InternalRulePriority=Speed  OutDataTypeStr=Inherit: Inherit from 'Table data'  RndMeth=Simplest
  EMTrq : Outport  VectorParamsAs1DForOutWhenUnconnected=off
  wires:
  EMSpd/1 -> MaxEMTrqVsSpd/1
  MaxEMTrqVsSpd/1 -> EMTrq/1

== system EvPowertrainController2EM/Accel Pedal to Traction Wheel Torque Request/EM2WhlTrq/3EM Dual Front/VehSpd2EMSpd ==
  Gear : Inport
  VehSpd : Inport  Port=2
  No Transmission : Subsystem  VariantControl=3
  Transmission : Subsystem  VariantControl=1
  EMSpdFrntAxl : Outport
  EMSpdRearAxl : Outport  Port=2

== system EvPowertrainController2EM/Accel Pedal to Traction Wheel Torque Request/EM2WhlTrq/3EM Dual Rear/EMTrq2WhlTrqFrnt ==
  Gear : Inport
  EMTrqCmd : Inport  Port=2
  EMSpd : Inport  Port=3
  No Transmission : Subsystem  VariantControl=3
  Transmission : Subsystem  VariantControl=1
  WhlMotTrq : Outport

== system EvPowertrainController2EM/Accel Pedal to Traction Wheel Torque Request/EM2WhlTrq/3EM Dual Rear/EMTrq2WhlTrqRear ==
  Gear : Inport
  EMTrqCmd : Inport  Port=2
  EMSpd : Inport  Port=3
  No Transmission : Subsystem  VariantControl=3
  Transmission : Subsystem  VariantControl=1
  WhlMotTrq : Outport

== system EvPowertrainController2EM/Accel Pedal to Traction Wheel Torque Request/EM2WhlTrq/3EM Dual Rear/Maximum Torque Front Axle ==
  EMSpd : Inport
  MaxEMTrqVsSpd : Lookup_n-D  NumberOfTableDimensions=1  BreakpointsForDimension1=PlntEM1Spd  Table=PlntEM1Trq  ExtrapMethod=Clip  UseLastTableValue=on  InternalRulePriority=Speed  OutDataTypeStr=Inherit: Inherit from 'Table data'  RndMeth=Simplest
  EMTrq : Outport  VectorParamsAs1DForOutWhenUnconnected=off
  wires:
  MaxEMTrqVsSpd/1 -> EMTrq/1
  EMSpd/1 -> MaxEMTrqVsSpd/1

== system EvPowertrainController2EM/Accel Pedal to Traction Wheel Torque Request/EM2WhlTrq/3EM Dual Rear/Maximum Torque Rear Axle ==
  EMSpd : Inport
  MaxEMTrqVsSpd : Lookup_n-D  NumberOfTableDimensions=1  BreakpointsForDimension1=PlntEM3Spd  Table=PlntEM3Trq  ExtrapMethod=Clip  UseLastTableValue=on  InternalRulePriority=Speed  OutDataTypeStr=Inherit: Inherit from 'Table data'  RndMeth=Simplest
  EMTrq : Outport  VectorParamsAs1DForOutWhenUnconnected=off
  wires:
  EMSpd/1 -> MaxEMTrqVsSpd/1
  MaxEMTrqVsSpd/1 -> EMTrq/1

== system EvPowertrainController2EM/Accel Pedal to Traction Wheel Torque Request/EM2WhlTrq/3EM Dual Rear/VehSpd2EMSpd ==
  Gear : Inport
  VehSpd : Inport  Port=2
  No Transmission : Subsystem  VariantControl=3
  Transmission : Subsystem  VariantControl=1
  EMSpdFrntAxl : Outport
  EMSpdRearAxl : Outport  Port=2

== system EvPowertrainController2EM/Accel Pedal to Traction Wheel Torque Request/EM2WhlTrq/4EM/EMTrq2WhlTrqFrnt ==
  Gear : Inport
  EMTrqCmd : Inport  Port=2
  EMSpd : Inport  Port=3
  No Transmission : Subsystem  VariantControl=3
  Transmission : Subsystem  VariantControl=1
  WhlMotTrq : Outport

== system EvPowertrainController2EM/Accel Pedal to Traction Wheel Torque Request/EM2WhlTrq/4EM/EMTrq2WhlTrqRear ==
  Gear : Inport
  EMTrqCmd : Inport  Port=2
  EMSpd : Inport  Port=3
  No Transmission : Subsystem  VariantControl=3
  Transmission : Subsystem  VariantControl=1
  WhlMotTrq : Outport

== system EvPowertrainController2EM/Accel Pedal to Traction Wheel Torque Request/EM2WhlTrq/4EM/Maximum Torque Front Axle ==
  EMSpd : Inport
  MaxEMTrqVsSpd : Lookup_n-D  NumberOfTableDimensions=1  BreakpointsForDimension1=PlntEM1Spd  Table=PlntEM1Trq  ExtrapMethod=Clip  UseLastTableValue=on  InternalRulePriority=Speed  OutDataTypeStr=Inherit: Inherit from 'Table data'  RndMeth=Simplest
  EMTrq : Outport  VectorParamsAs1DForOutWhenUnconnected=off
  wires:
  EMSpd/1 -> MaxEMTrqVsSpd/1
  MaxEMTrqVsSpd/1 -> EMTrq/1

== system EvPowertrainController2EM/Accel Pedal to Traction Wheel Torque Request/EM2WhlTrq/4EM/Maximum Torque Rear Axle ==
  EMSpd : Inport
  MaxEMTrqVsSpd : Lookup_n-D  NumberOfTableDimensions=1  BreakpointsForDimension1=PlntEM3Spd  Table=PlntEM3Trq  ExtrapMethod=Clip  UseLastTableValue=on  InternalRulePriority=Speed  OutDataTypeStr=Inherit: Inherit from 'Table data'  RndMeth=Simplest
  EMTrq : Outport  VectorParamsAs1DForOutWhenUnconnected=off
  wires:
  MaxEMTrqVsSpd/1 -> EMTrq/1
  EMSpd/1 -> MaxEMTrqVsSpd/1

== system EvPowertrainController2EM/Accel Pedal to Traction Wheel Torque Request/EM2WhlTrq/4EM/VehSpd2EMSpd ==
  Gear : Inport
  VehSpd : Inport  Port=2
  No Transmission : Subsystem  VariantControl=3
  Transmission : Subsystem  VariantControl=1
  EMSpdFrntAxl : Outport
  EMSpdRearAxl : Outport  Port=2

== system EvPowertrainController2EM/Energy Management/Calculate Average EMSpd and Wheel Torque Curves for Front and Rear Axles/2EM/EMTrq2WhlTrqFrnt ==
  Gear : Inport
  EMTrqCmd : Inport  Port=2
  EMSpd : Inport  Port=3
  No Transmission : Subsystem  VariantControl=3
  Transmission : Subsystem  VariantControl=1
  WhlMotTrq : Outport

== system EvPowertrainController2EM/Energy Management/Calculate Average EMSpd and Wheel Torque Curves for Front and Rear Axles/2EM/EMTrq2WhlTrqRear ==
  Gear : Inport
  EMTrqCmd : Inport  Port=2
  EMSpd : Inport  Port=3
  No Transmission : Subsystem  VariantControl=3
  Transmission : Subsystem  VariantControl=1
  WhlMotTrq : Outport

== system EvPowertrainController2EM/Energy Management/Calculate Average EMSpd and Wheel Torque Curves for Front and Rear Axles/2EM/Maximum Torque Front Axle ==
  EMSpd : Inport
  MaxEMTrqVsSpd : Lookup_n-D  NumberOfTableDimensions=1  BreakpointsForDimension1=PlntEM1Spd  Table=PlntEM1Trq  ExtrapMethod=Clip  UseLastTableValue=on  InternalRulePriority=Speed  OutDataTypeStr=Inherit: Inherit from 'Table data'  RndMeth=Simplest
  EMTrq : Outport  VectorParamsAs1DForOutWhenUnconnected=off
  wires:
  MaxEMTrqVsSpd/1 -> EMTrq/1
  EMSpd/1 -> MaxEMTrqVsSpd/1

== system EvPowertrainController2EM/Energy Management/Calculate Average EMSpd and Wheel Torque Curves for Front and Rear Axles/2EM/Maximum Torque Rear Axle ==
  EMSpd : Inport
  MaxEMTrqVsSpd : Lookup_n-D  NumberOfTableDimensions=1  BreakpointsForDimension1=PlntEM2Spd  Table=PlntEM2Trq  ExtrapMethod=Clip  UseLastTableValue=on  InternalRulePriority=Speed  OutDataTypeStr=Inherit: Inherit from 'Table data'  RndMeth=Simplest
  EMTrq : Outport  VectorParamsAs1DForOutWhenUnconnected=off
  wires:
  MaxEMTrqVsSpd/1 -> EMTrq/1
  EMSpd/1 -> MaxEMTrqVsSpd/1

== system EvPowertrainController2EM/Energy Management/Calculate Average EMSpd and Wheel Torque Curves for Front and Rear Axles/3EM Dual Front/EMTrq2WhlTrqFrnt ==
  Gear : Inport
  EMTrqCmd : Inport  Port=2
  EMSpd : Inport  Port=3
  No Transmission : Subsystem  VariantControl=3
  Transmission : Subsystem  VariantControl=1
  WhlMotTrq : Outport

== system EvPowertrainController2EM/Energy Management/Calculate Average EMSpd and Wheel Torque Curves for Front and Rear Axles/3EM Dual Front/EMTrq2WhlTrqRear ==
  Gear : Inport
  EMTrqCmd : Inport  Port=2
  EMSpd : Inport  Port=3
  No Transmission : Subsystem  VariantControl=3
  Transmission : Subsystem  VariantControl=1
  WhlMotTrq : Outport

== system EvPowertrainController2EM/Energy Management/Calculate Average EMSpd and Wheel Torque Curves for Front and Rear Axles/3EM Dual Front/Maximum Torque Front Axle ==
  EMSpd : Inport
  MaxEMTrqVsSpd : Lookup_n-D  NumberOfTableDimensions=1  BreakpointsForDimension1=PlntEM1Spd  Table=PlntEM1Trq  ExtrapMethod=Clip  UseLastTableValue=on  InternalRulePriority=Speed  OutDataTypeStr=Inherit: Inherit from 'Table data'  RndMeth=Simplest
  EMTrq : Outport  VectorParamsAs1DForOutWhenUnconnected=off
  wires:
  EMSpd/1 -> MaxEMTrqVsSpd/1
  MaxEMTrqVsSpd/1 -> EMTrq/1

== system EvPowertrainController2EM/Energy Management/Calculate Average EMSpd and Wheel Torque Curves for Front and Rear Axles/3EM Dual Front/Maximum Torque Rear Axle ==
  EMSpd : Inport
  MaxEMTrqVsSpd : Lookup_n-D  NumberOfTableDimensions=1  BreakpointsForDimension1=PlntEM3Spd  Table=PlntEM3Trq  ExtrapMethod=Clip  UseLastTableValue=on  InternalRulePriority=Speed  OutDataTypeStr=Inherit: Inherit from 'Table data'  RndMeth=Simplest
  EMTrq : Outport  VectorParamsAs1DForOutWhenUnconnected=off
  wires:
  EMSpd/1 -> MaxEMTrqVsSpd/1
  MaxEMTrqVsSpd/1 -> EMTrq/1

== system EvPowertrainController2EM/Energy Management/Calculate Average EMSpd and Wheel Torque Curves for Front and Rear Axles/3EM Dual Rear/EMTrq2WhlTrqFrnt ==
  Gear : Inport
  EMTrqCmd : Inport  Port=2
  EMSpd : Inport  Port=3
  No Transmission : Subsystem  VariantControl=3
  Transmission : Subsystem  VariantControl=1
  WhlMotTrq : Outport

== system EvPowertrainController2EM/Energy Management/Calculate Average EMSpd and Wheel Torque Curves for Front and Rear Axles/3EM Dual Rear/EMTrq2WhlTrqRear ==
  Gear : Inport
  EMTrqCmd : Inport  Port=2
  EMSpd : Inport  Port=3
  No Transmission : Subsystem  VariantControl=3
  Transmission : Subsystem  VariantControl=1
  WhlMotTrq : Outport

== system EvPowertrainController2EM/Energy Management/Calculate Average EMSpd and Wheel Torque Curves for Front and Rear Axles/3EM Dual Rear/Maximum Torque Front Axle ==
  EMSpd : Inport
  MaxEMTrqVsSpd : Lookup_n-D  NumberOfTableDimensions=1  BreakpointsForDimension1=PlntEM1Spd  Table=PlntEM1Trq  ExtrapMethod=Clip  UseLastTableValue=on  InternalRulePriority=Speed  OutDataTypeStr=Inherit: Inherit from 'Table data'  RndMeth=Simplest
  EMTrq : Outport  VectorParamsAs1DForOutWhenUnconnected=off
  wires:
  MaxEMTrqVsSpd/1 -> EMTrq/1
  EMSpd/1 -> MaxEMTrqVsSpd/1

== system EvPowertrainController2EM/Energy Management/Calculate Average EMSpd and Wheel Torque Curves for Front and Rear Axles/3EM Dual Rear/Maximum Torque Rear Axle ==
  EMSpd : Inport
  MaxEMTrqVsSpd : Lookup_n-D  NumberOfTableDimensions=1  BreakpointsForDimension1=PlntEM3Spd  Table=PlntEM3Trq  ExtrapMethod=Clip  UseLastTableValue=on  InternalRulePriority=Speed  OutDataTypeStr=Inherit: Inherit from 'Table data'  RndMeth=Simplest
  EMTrq : Outport  VectorParamsAs1DForOutWhenUnconnected=off
  wires:
  EMSpd/1 -> MaxEMTrqVsSpd/1
  MaxEMTrqVsSpd/1 -> EMTrq/1

== system EvPowertrainController2EM/Energy Management/Calculate Average EMSpd and Wheel Torque Curves for Front and Rear Axles/4EM/EMTrq2WhlTrqFrnt ==
  Gear : Inport
  EMTrqCmd : Inport  Port=2
  EMSpd : Inport  Port=3
  No Transmission : Subsystem  VariantControl=3
  Transmission : Subsystem  VariantControl=1
  WhlMotTrq : Outport

== system EvPowertrainController2EM/Energy Management/Calculate Average EMSpd and Wheel Torque Curves for Front and Rear Axles/4EM/EMTrq2WhlTrqRear ==
  Gear : Inport
  EMTrqCmd : Inport  Port=2
  EMSpd : Inport  Port=3
  No Transmission : Subsystem  VariantControl=3
  Transmission : Subsystem  VariantControl=1
  WhlMotTrq : Outport

== system EvPowertrainController2EM/Energy Management/Calculate Average EMSpd and Wheel Torque Curves for Front and Rear Axles/4EM/Maximum Torque Front Axle ==
  EMSpd : Inport
  MaxEMTrqVsSpd : Lookup_n-D  NumberOfTableDimensions=1  BreakpointsForDimension1=PlntEM1Spd  Table=PlntEM1Trq  ExtrapMethod=Clip  UseLastTableValue=on  InternalRulePriority=Speed  OutDataTypeStr=Inherit: Inherit from 'Table data'  RndMeth=Simplest
  EMTrq : Outport  VectorParamsAs1DForOutWhenUnconnected=off
  wires:
  EMSpd/1 -> MaxEMTrqVsSpd/1
  MaxEMTrqVsSpd/1 -> EMTrq/1

== system EvPowertrainController2EM/Energy Management/Calculate Average EMSpd and Wheel Torque Curves for Front and Rear Axles/4EM/Maximum Torque Rear Axle ==
  EMSpd : Inport
  MaxEMTrqVsSpd : Lookup_n-D  NumberOfTableDimensions=1  BreakpointsForDimension1=PlntEM3Spd  Table=PlntEM3Trq  ExtrapMethod=Clip  UseLastTableValue=on  InternalRulePriority=Speed  OutDataTypeStr=Inherit: Inherit from 'Table data'  RndMeth=Simplest
  EMTrq : Outport  VectorParamsAs1DForOutWhenUnconnected=off
  wires:
  MaxEMTrqVsSpd/1 -> EMTrq/1
  EMSpd/1 -> MaxEMTrqVsSpd/1

== system EvPowertrainController2EM/Energy Management/Control Domain /Front Axle EM Torque Vector/2EM or 3EM Dual Rear ==
  EMAvgSpdVec : Inport
  Diff Eta : Subsystem
  Divide2 : Product  Inputs=**
  EMTrq Control Vector Traction : Constant  Value=linspace(0, max(PlntEM1Trq), CtrlVcuEMTrqSplitGrid)  SampleTime=-1
  Gain : Gain  Gain=-1
  Gain3 : Gain  Gain=PlntDiffrntlRatio
  Selector : Selector  InputPortWidth=2  IndexOptions=Index vector (dialog)  Indices=[1]  OutputSizes=1
  WhlEMFrntVecPos : Outport
  WhlEMFrntVecNeg : Outport  Port=2
  wires:
  Selector/1 -> Diff Eta/1(SpdIn)
  Gain3/1 -> Divide2/2
  Diff Eta/1(eta) -> Divide2/1
  Divide2/1 -> WhlEMFrntVecPos/1, Gain/1
  EMTrq Control Vector Traction/1 -> Gain3/1, Diff Eta/2(TrqIn)
  EMAvgSpdVec/1 -> Selector/1
  Gain/1 -> WhlEMFrntVecNeg/1

== system EvPowertrainController2EM/Energy Management/Control Domain /Front Axle EM Torque Vector/3EM Dual Front or 4EM ==
  EMAvgSpdVec : Inport
  Divide2 : Product  Inputs=**
  Dual EMs : Gain  Gain=2
  EMTrq Control Vector Traction : Constant  Value=linspace(0, max(PlntEM1Trq), CtrlVcuEMTrqSplitGrid)  SampleTime=-1
  Gain : Gain  Gain=-1
  Gain3 : Gain  Gain=PlntEMWhlGearRatioFL
  Gear Eta : Subsystem
  Selector : Selector  InputPortWidth=2  IndexOptions=Index vector (dialog)  Indices=[1]  OutputSizes=1
  WhlEMFrntVecPos : Outport
  WhlEMFrntVecNeg : Outport  Port=2
  wires:
  Selector/1 -> Gear Eta/1(SpdIn)
  Gain/1 -> WhlEMFrntVecNeg/1
  Divide2/1 -> WhlEMFrntVecPos/1, Gain/1
  Gear Eta/1(eta) -> Divide2/1
  Dual EMs/1 -> Gear Eta/2(TrqIn), Gain3/1
  EMTrq Control Vector Traction/1 -> Dual EMs/1
  EMAvgSpdVec/1 -> Selector/1
  Gain3/1 -> Divide2/2

== system EvPowertrainController2EM/Energy Management/Control Domain /Rear Axle EM Torque Vector/2EM or 3EM Dual Front ==
  EMAvgSpdVec : Inport
  Diff Eta : Subsystem
  Divide2 : Product  Inputs=**
  EMTrq Control Vector Traction : Constant  Value=linspace(0, max(PlntEM2Trq), CtrlVcuEMTrqSplitGrid)  SampleTime=-1
  Gain : Gain  Gain=-1
  Gain3 : Gain  Gain=PlntDiffrntl2Ratio
  Selector : Selector  InputPortWidth=2  IndexOptions=Index vector (dialog)  Indices=[2]  OutputSizes=1
  WhlEMRearVecPos : Outport
  WhlEMRearVecNeg : Outport  Port=2
  wires:
  Gain/1 -> WhlEMRearVecNeg/1
  EMAvgSpdVec/1 -> Selector/1
  EMTrq Control Vector Traction/1 -> Diff Eta/2(TrqIn), Gain3/1
  Divide2/1 -> Gain/1, WhlEMRearVecPos/1
  Diff Eta/1(eta) -> Divide2/1
  Gain3/1 -> Divide2/2
  Selector/1 -> Diff Eta/1(SpdIn)

== system EvPowertrainController2EM/Energy Management/Control Domain /Rear Axle EM Torque Vector/3EM Dual Rear or 4EM ==
  EMAvgSpdVec : Inport
  Divide2 : Product  Inputs=**
  Dual EMs : Gain  Gain=2
  EMTrq Control Vector Traction : Constant  Value=linspace(0, max(PlntEM3Trq), CtrlVcuEMTrqSplitGrid)  SampleTime=-1
  Gain : Gain  Gain=-1
  Gain3 : Gain  Gain=PlntEMWhlGearRatioRL
  Gear Eta : Subsystem
  Selector : Selector  InputPortWidth=2  IndexOptions=Index vector (dialog)  Indices=[2]  OutputSizes=1
  WhlEMRearVecPos : Outport
  WhlEMRearVecNeg : Outport  Port=2
  wires:
  Gain3/1 -> Divide2/2
  EMAvgSpdVec/1 -> Selector/1
  EMTrq Control Vector Traction/1 -> Dual EMs/1
  Dual EMs/1 -> Gain3/1, Gear Eta/2(TrqIn)
  Gear Eta/1(eta) -> Divide2/1
  Divide2/1 -> Gain/1, WhlEMRearVecPos/1
  Gain/1 -> WhlEMRearVecNeg/1
  Selector/1 -> Gear Eta/1(SpdIn)

== system EvPowertrainController2EM/Energy Management/Convert Whl to EMTrq Vector/2EM/Diff Eta ==
  note: Pwr >= 0, v = 1
      | Pwr < 0, v= -1
  SpdIn : Inport
  TrqIn : Inport  Port=2
  Constant : Constant  Value=PlntDiffrntlEff
  Constant1 : Constant  SampleTime=-1
  Constant2 : Constant  Value=-1  SampleTime=-1
  Math Function1 : Math  Operator=pow  SignedPower=on  OutputSignalType=real
  Product1 : Product
  Switch2 : Switch  SaturateOnIntegerOverflow=off  InputSameDT=off
  eta : Outport  VectorParamsAs1DForOutWhenUnconnected=off
  wires:
  SpdIn/1 -> Product1/2
  Constant/1 -> Math Function1/1
  Constant2/1 -> Switch2/3
  Constant1/1 -> Switch2/1
  Product1/1 -> Switch2/2
  Switch2/1 -> Math Function1/2
  Math Function1/1 -> eta/1
  TrqIn/1 -> Product1/1

== system EvPowertrainController2EM/Energy Management/Convert Whl to EMTrq Vector/2EM/Diff Eta1 ==
  note: Pwr >= 0, v = 1
      | Pwr < 0, v= -1
  SpdIn : Inport
  TrqIn : Inport  Port=2
  Constant : Constant  Value=PlntDiffrntl2Eff
  Constant1 : Constant  SampleTime=-1
  Constant2 : Constant  Value=-1  SampleTime=-1
  Math Function1 : Math  Operator=pow  SignedPower=on  OutputSignalType=real
  Product1 : Product
  Switch2 : Switch  SaturateOnIntegerOverflow=off  InputSameDT=off
  eta : Outport  VectorParamsAs1DForOutWhenUnconnected=off
  wires:
  TrqIn/1 -> Product1/1
  Math Function1/1 -> eta/1
  Switch2/1 -> Math Function1/2
  Product1/1 -> Switch2/2
  Constant1/1 -> Switch2/1
  Constant2/1 -> Switch2/3
  Constant/1 -> Math Function1/1
  SpdIn/1 -> Product1/2

== system EvPowertrainController2EM/Energy Management/Convert Whl to EMTrq Vector/3EM Dual Front/Diff Eta ==
  note: Pwr >= 0, v = 1
      | Pwr < 0, v= -1
  SpdIn : Inport
  TrqIn : Inport  Port=2
  Constant : Constant  Value=PlntDiffrntl2Eff
  Constant1 : Constant  SampleTime=-1
  Constant2 : Constant  Value=-1  SampleTime=-1
  Math Function1 : Math  Operator=pow  SignedPower=on  OutputSignalType=real
  Product1 : Product
  Switch2 : Switch  SaturateOnIntegerOverflow=off  InputSameDT=off
  eta : Outport  VectorParamsAs1DForOutWhenUnconnected=off
  wires:
  SpdIn/1 -> Product1/2
  Constant/1 -> Math Function1/1
  Constant2/1 -> Switch2/3
  Constant1/1 -> Switch2/1
  Product1/1 -> Switch2/2
  Switch2/1 -> Math Function1/2
  Math Function1/1 -> eta/1
  TrqIn/1 -> Product1/1

== system EvPowertrainController2EM/Energy Management/Convert Whl to EMTrq Vector/3EM Dual Front/Gear Eta ==
  note: Pwr >= 0, v = 1
      | Pwr < 0, v= -1
  SpdIn : Inport
  TrqIn : Inport  Port=2
  Constant : Constant  Value=PlntEMWhlGearEffFL
  Constant1 : Constant  SampleTime=-1
  Constant2 : Constant  Value=-1  SampleTime=-1
  Math Function1 : Math  Operator=pow  SignedPower=on  OutputSignalType=real
  Product1 : Product
  Switch2 : Switch  SaturateOnIntegerOverflow=off  InputSameDT=off
  eta : Outport  VectorParamsAs1DForOutWhenUnconnected=off
  wires:
  TrqIn/1 -> Product1/1
  Math Function1/1 -> eta/1
  Switch2/1 -> Math Function1/2
  Product1/1 -> Switch2/2
  Constant1/1 -> Switch2/1
  Constant2/1 -> Switch2/3
  Constant/1 -> Math Function1/1
  SpdIn/1 -> Product1/2

== system EvPowertrainController2EM/Energy Management/Convert Whl to EMTrq Vector/3EM Dual Rear/Diff Eta ==
  note: Pwr >= 0, v = 1
      | Pwr < 0, v= -1
  SpdIn : Inport
  TrqIn : Inport  Port=2
  Constant : Constant  Value=PlntDiffrntlEff
  Constant1 : Constant  SampleTime=-1
  Constant2 : Constant  Value=-1  SampleTime=-1
  Math Function1 : Math  Operator=pow  SignedPower=on  OutputSignalType=real
  Product1 : Product
  Switch2 : Switch  SaturateOnIntegerOverflow=off  InputSameDT=off
  eta : Outport  VectorParamsAs1DForOutWhenUnconnected=off
  wires:
  SpdIn/1 -> Product1/2
  Constant/1 -> Math Function1/1
  Constant2/1 -> Switch2/3
  Constant1/1 -> Switch2/1
  Product1/1 -> Switch2/2
  Switch2/1 -> Math Function1/2
  Math Function1/1 -> eta/1
  TrqIn/1 -> Product1/1

== system EvPowertrainController2EM/Energy Management/Convert Whl to EMTrq Vector/3EM Dual Rear/Gear Eta ==
  note: Pwr >= 0, v = 1
      | Pwr < 0, v= -1
  SpdIn : Inport
  TrqIn : Inport  Port=2
  Constant : Constant  Value=PlntEMWhlGearEffRL
  Constant1 : Constant  SampleTime=-1
  Constant2 : Constant  Value=-1  SampleTime=-1
  Math Function1 : Math  Operator=pow  SignedPower=on  OutputSignalType=real
  Product1 : Product
  Switch2 : Switch  SaturateOnIntegerOverflow=off  InputSameDT=off
  eta : Outport  VectorParamsAs1DForOutWhenUnconnected=off
  wires:
  TrqIn/1 -> Product1/1
  Math Function1/1 -> eta/1
  Switch2/1 -> Math Function1/2
  Product1/1 -> Switch2/2
  Constant1/1 -> Switch2/1
  Constant2/1 -> Switch2/3
  Constant/1 -> Math Function1/1
  SpdIn/1 -> Product1/2

== system EvPowertrainController2EM/Energy Management/Convert Whl to EMTrq Vector/4EM/Gear Eta ==
  note: Pwr >= 0, v = 1
      | Pwr < 0, v= -1
  SpdIn : Inport
  TrqIn : Inport  Port=2
  Constant : Constant  Value=PlntEMWhlGearEffFL
  Constant1 : Constant  SampleTime=-1
  Constant2 : Constant  Value=-1  SampleTime=-1
  Math Function1 : Math  Operator=pow  SignedPower=on  OutputSignalType=real
  Product1 : Product
  Switch2 : Switch  SaturateOnIntegerOverflow=off  InputSameDT=off
  eta : Outport  VectorParamsAs1DForOutWhenUnconnected=off
  wires:
  TrqIn/1 -> Product1/1
  Math Function1/1 -> eta/1
  Switch2/1 -> Math Function1/2
  Product1/1 -> Switch2/2
  Constant1/1 -> Switch2/1
  Constant2/1 -> Switch2/3
  Constant/1 -> Math Function1/1
  SpdIn/1 -> Product1/2
